simulink model "simulinkDiscretePID"  (R2021a)
settings: Solver=VariableStepAuto  StartTime=0.0  StopTime=500.0  RelTol=1e-3
values from neighbouring files (symbols this model uses):
  Ad = sysd.a    [main.m]    (also in prova_Esame.m)
  Bd = sysd.b    [main.m]    (also in prova_Esame.m)
  C = [0 0 1 0]    [main.m]    (also in prova_Esame.m = [0, 0, 1, 0])
  D = zeros(1,1)    [main.m]    (also in prova_Esame.m)
  sampleTime = 0.1    [main.m]    (also in prova_Esame.m)
  x0 = [0 0 0 0]'    [main.m]    (also in prova_Esame.m)
libraries: pid_lib x1
settings Model: Creator=miren  LastModifiedBy=marco

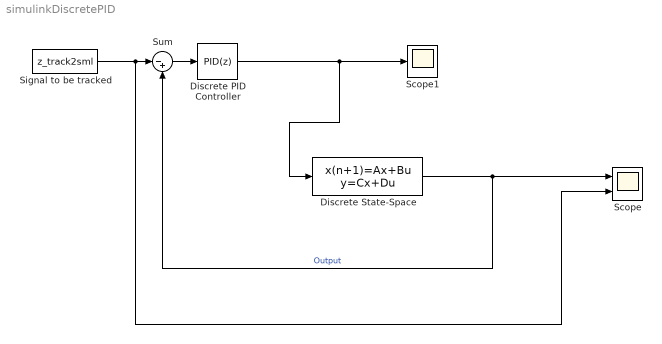
== system simulinkDiscretePID ==
  Discrete PID Controller : pid_lib/PID Controller  Controller=PID  Form=Parallel  TimeDomain=Discrete-time  UseExternalTs=off  SampleTime=sampleTime  IntegratorMethod=Forward Euler  FilterMethod=Forward Euler  ControllerParametersSource=internal  P=-0.263603490582703  I=-0.00167453358790764  D=-9.24659049240749  UseFilter=on  N=0.373913366788932  TunerSelectOption=Transfer Function Based (PID Tuner App)  InitialConditionSource=internal  InitialConditionForIntegrator=0  InitialConditionForFilter=0  DifferentiatorICPrevScaledInput=0  ExternalReset=none  TrackingMode=off  Kt=1  LimitOutput=off  SatLimitsSource=internal  UpperSaturationLimit=1000  LowerSaturationLimit=0  LinearizeAsGain=off  AntiWindupMode=clamping  Kb=1  POutMin=[]  POutMax=[]  IOutMin=[]  IOutMax=[]  DOutMin=[]  DOutMax=[]  NOutMin=[]  NOutMax=[]  SumOutMin=[]  SumOutMax=[]  SaturationOutMin=[]  SaturationOutMax=[]  PParamMin=[]  PParamMax=[]  IParamMin=[]  IParamMax=[]  DParamMin=[]  DParamMax=[]  NParamMin=[]  NParamMax=[]  KbParamMin=[]  KbParamMax=[]  KtParamMin=[]  KtParamMax=[]  KbOutMin=[]  KbOutMax=[]  KtOutMin=[]  KtOutMax=[]  IntegratorOutMin=[]  IntegratorOutMax=[]  FilterOutMin=[]  FilterOutMax=[]  SumI1OutMin=[]  SumI1OutMax=[]  SumI2OutMin=[]  SumI2OutMax=[]  SumI3OutMin=[]  SumI3OutMax=[]  SumI4OutMin=[]  SumI4OutMax=[]  SumDOutMin=[]  SumDOutMax=[]  DifferentiatorOutMin=[]  DifferentiatorOutMax=[]  FilterDiffOutCoefMin=[]  FilterDiffOutCoefMax=[]  ReciprocalOutMin=[]  ReciprocalOutMax=[]  SumDenOutMin=[]  SumDenOutMax=[]  SumNumOutMin=[]  SumNumOutMax=[]  DivideOutMin=[]  DivideOutMax=[]  UdiffTsProdOutMin=[]  UdiffTsProdOutMax=[]  NTsProdOutMin=[]  NTsProdOutMax=[]  UintegralTsProdOutMin=[]  UintegralTsProdOutMax=[]  UngainTsProdOutMin=[]  UngainTsProdOutMax=[]  IntegratorContinuousStateAttributes=''  IntegratorStateMustResolveToSignalObject=off  IntegratorRTWStateStorageClass=Auto  FilterContinuousStateAttributes=''  FilterStateMustResolveToSignalObject=off  FilterRTWStateStorageClass=Auto  ParallelPVariant=InternalParameters  IdealPVariant=Disabled  IVariant=InternalParameters  DVariant=InternalParameters  IntegratorVariant=Discrete  SatVariant=Disabled  AWVariant=Passthrough  PCopyVariant=Disabled  TRVariant=Disabled  FdbkBlocksVariant=Forward  IdealPFdbkVariant=Disabled  SatFdbkVariant=Disabled  DerivativeFilterVariant=ForwardEulerFilter  NVariant=InternalParameters  NCopyVariant=Disabled  FilterICVariant=InternalICsFilter  IntegratorICVariant=InternalICs  ExternalResetVariant=Disabled  TRSumVariant=Passthrough  SumFdbkVariant=Disabled  SumVariant=Sum_PID  TsampFilterVariant=InternalTs  TsampNgainVariant=Passthrough  TsampIntegralVariant=Passthrough  ExternalSaturationOutDataTypeStr=Inherit: Same as second input
  Discrete State-Space : DiscreteStateSpace  A=Ad  B=Bd  C=C  D=D  InitialCondition=x0  SampleTime=sampleTime
  Scope : Scope  NumInputPorts=2
  Scope1 : Scope
  "Signal to be tracked " : FromWorkspace  VariableName=z_track2sml  SampleTime=sampleTime
  Sum : Sum  Inputs=|-+
  wires:
  Sum/1 -> Discrete PID Controller/1
  "Signal to be tracked "/1 -> Scope/2, Sum/1
  Discrete State-Space/1 -> Scope/1, Sum/2  "Output"
  Discrete PID Controller/1 -> Discrete State-Space/1, Scope1/1
